simulink model "sim_battery_pack_simulink_18_11"  (R2021a)
settings: Solver=FixedStepAuto  StartTime=0.0  StopTime=3460.480  FixedStep=0.01  RelTol=1e-3
values from neighbouring files (symbols this model uses):
  Af = 1.4*1.6    (= 2.24)    [battery_pack_init_18_11.m]
  b = 0.002    [battery_pack_init_18_11.m]
  Batt_Eff = .98    (= 0.98)    [battery_pack_init_18_11.m]
  Batt_Ene_Cap = 7.37    [battery_pack_init_18_11.m]
  cd = 0.45    [battery_pack_init_18_11.m]
  dt = 0.01    [battery_pack_init_18_11.m]
  g = 9.81    [battery_pack_init_18_11.m]
  Gr = 5.75*.85    (= 4.8875)    [battery_pack_init_18_11.m]
  Grade = 7    [battery_pack_init_18_11.m]
  Ini_SOC = 100    [battery_pack_init_18_11.m]
  kappa = 0.1    [battery_pack_init_18_11.m]
  M = M_k+M_P    (= 445)    [battery_pack_init_18_11.m]
  M_Trq = T_m    [battery_pack_init_18_11.m]
  M_w = w_m    [battery_pack_init_18_11.m]
  Mot_Eff = .9    (= 0.9)    [battery_pack_init_18_11.m]
  mu = 0.016    [battery_pack_init_18_11.m]
  Np = 7    [battery_pack_init_18_11.m]
  Ns = 12    [battery_pack_init_18_11.m]
  Qgain = 1    [battery_pack_init_18_11.m]
  R0 = zeros(numpoles,1)    [battery_pack_init_18_11.m]
  R0Param = getParamESC('R0Param',T,cell_model)    [battery_pack_init_18_11.m]
  R_w = .3048/2    (= 0.1524)    [battery_pack_init_18_11.m]
  Re_spe_max = 50*5/18    (= 13.8888888889)    [battery_pack_init_18_11.m]
  Re_spe_min = 0*5/18    (= 0)    [battery_pack_init_18_11.m]
  rho = 1.225    [battery_pack_init_18_11.m]
  rt = .0008    (= 0.0008)    [battery_pack_init_18_11.m]
  T = 40    [battery_pack_init_18_11.m]
  T_MIDC = T_MIDC(1:72)    [battery_pack_init_18_11.m]
  Trans_Eff = .95    (= 0.95)    [battery_pack_init_18_11.m]
  V_MIDC = V_MIDC(1:72)    [battery_pack_init_18_11.m]
  Z0 = 0.75 + (1-0.75).*rand(1,Np)    [battery_pack_init_18_11.m]
undefined symbols (not defined in the file or in its folder): cell_model, FLbattery, gain, iload, sigbuilder_block, VMIDC
libraries: simulink x16, autolibshared x2, pid_lib x1, simulink_extras x1
(part 1 of 17)
settings Model: Creator=User  LastModifiedBy=User

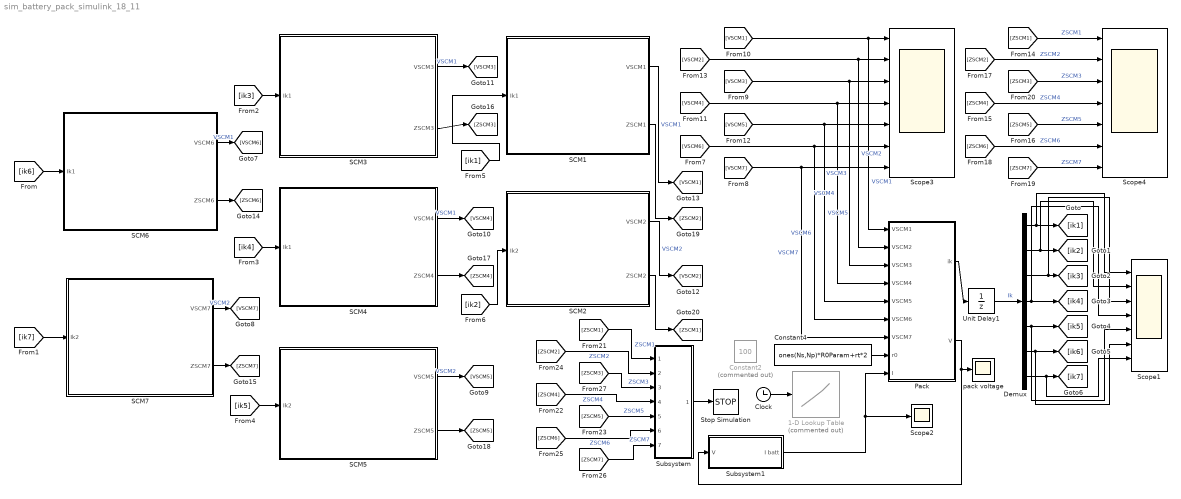
== system sim_battery_pack_simulink_18_11 ==
  1-D Lookup Table : Lookup_n-D  Commented=on  NumberOfTableDimensions=1  BreakpointsForDimension1=0:0.01:3460.480  Table=iload  InternalRulePriority=Speed  RndMeth=Simplest  InputSameDT=on
  Clock : Clock
  Constant2 : Constant  Commented=on  Value=100
  Constant4 : Constant  Value=ones(Ns,Np)*R0Param+rt*2
  Demux : Demux  Outputs=7
  Pack : MATLAB Function  TreatAsAtomicUnit=on
  SCM1 : Subsystem
  SCM2 : Subsystem
  SCM3 : Subsystem
  SCM4 : Subsystem
  SCM5 : Subsystem
  SCM6 : Subsystem
  SCM7 : Subsystem
  Scope1 : Scope  NumInputPorts=7
  Scope2 : Scope
  Scope3 : Scope  NumInputPorts=7
  Scope4 : Scope  NumInputPorts=7
  Stop Simulation : Stop
  Subsystem : Subsystem
  Subsystem1 : Subsystem
  Unit Delay1 : UnitDelay  SampleTime=-1  HasFrameUpgradeWarning=on
  pack voltage : Scope
  wires:
  Subsystem1/1(I batt) -> Pack/9(I), Scope2/1
  [VSCM1] -> Pack/1(VSCM1), Scope3/1  "VSCM1"
  [VSCM2] -> Scope3/2, Pack/2(VSCM2)  "VSCM2"
  Pack/1(ik) -> Unit Delay1/1
  Unit Delay1/1 -> Demux/1  "Ik"
  Constant4/1 -> Pack/8(r0)
  Clock/1 -> 1-D Lookup Table/1
  [VSCM3] -> Scope3/3, Pack/3(VSCM3)  "VSCM3"
  [VSCM4] -> Pack/4(VSCM4), Scope3/4  "VSCM4"
  [VSCM5] -> Pack/5(VSCM5), Scope3/5  "VSCM5"
  [VSCM6] -> Pack/6(VSCM6), Scope3/6  "VSCM6"
  [VSCM7] -> Scope3/7, Pack/7(VSCM7)  "VSCM7"
  [ik7] -> SCM7/1(Ik2)
  [ik6] -> SCM6/1(Ik1)
  [ik3] -> SCM3/1(Ik1)
  [ik4] -> SCM4/1(Ik1)
  [ik5] -> SCM5/1(Ik2)
  [ik2] -> SCM2/1(Ik2)
  [ik1] -> SCM1/1(Ik1)
  Demux/1 -> Scope1/1, [ik1]
  Demux/2 -> [ik2], Scope1/2
  Demux/3 -> Scope1/3, [ik3]
  Demux/4 -> [ik4], Scope1/4
  Demux/5 -> [ik5], Scope1/5
  Demux/6 -> [ik6], Scope1/6
  Demux/7 -> Scope1/7, [ik7]
  SCM6/1(VSCM6) -> [VSCM6]  "VSCM1"
  SCM7/1(VSCM7) -> [VSCM7]  "VSCM2"
  SCM1/1(VSCM1) -> [VSCM1]  "VSCM1"
  SCM2/1(VSCM2) -> [VSCM2]  "VSCM2"
  SCM5/1(VSCM5) -> [VSCM5]  "VSCM2"
  SCM4/1(VSCM4) -> [VSCM4]  "VSCM1"
  SCM3/1(VSCM3) -> [VSCM3]  "VSCM1"
  Pack/2(V) -> Subsystem1/1(V), pack voltage/1
  SCM6/2(ZSCM6) -> [ZSCM6]
  SCM7/2(ZSCM7) -> [ZSCM7]
  SCM3/2(ZSCM3) -> [ZSCM3]
  SCM4/2(ZSCM4) -> [ZSCM4]
  SCM5/2(ZSCM5) -> [ZSCM5]
  SCM1/2(ZSCM1) -> [ZSCM2]
  SCM2/2(ZSCM2) -> [ZSCM1]
  [ZSCM7] -> Scope4/7  "ZSCM7"
  [ZSCM6] -> Scope4/6  "ZSCM6"
  [ZSCM5] -> Scope4/5  "ZSCM5"
  [ZSCM4] -> Scope4/4  "ZSCM4"
  [ZSCM3] -> Scope4/3  "ZSCM3"
  [ZSCM2] -> Scope4/2  "ZSCM2"
  [ZSCM1] -> Scope4/1  "ZSCM1"
  [ZSCM2] -> Subsystem/2(ZSCM2)  "ZSCM2"
  [ZSCM4] -> Subsystem/4(ZSCM4)  "ZSCM4"
  [ZSCM6] -> Subsystem/6(ZSCM6)  "ZSCM6"
  [ZSCM1] -> Subsystem/1(ZSCM1)  "ZSCM1"
  [ZSCM3] -> Subsystem/3(ZSCM3)  "ZSCM3"
  [ZSCM5] -> Subsystem/5(ZSCM5)  "ZSCM5"
  [ZSCM7] -> Subsystem/7(ZSCM7)  "ZSCM7"
  Subsystem/1(STOP) -> Stop Simulation/1

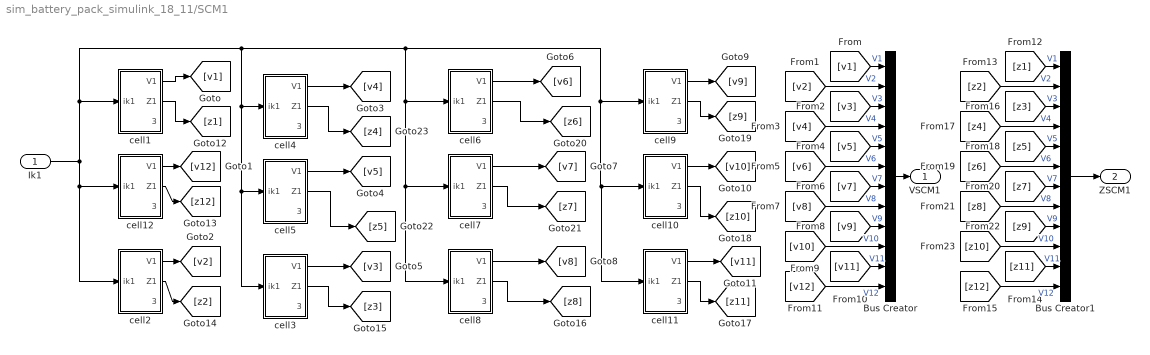
== system sim_battery_pack_simulink_18_11/SCM1 ==
  Ik1 : Inport
  Bus Creator : BusCreator  Inputs=12
  Bus Creator1 : BusCreator  Inputs=12
  cell1 : Subsystem
  cell10 : Subsystem
  cell11 : Subsystem
  cell12 : Subsystem
  cell2 : Subsystem
  cell3 : Subsystem
  cell4 : Subsystem
  cell5 : Subsystem
  cell6 : Subsystem
  cell7 : Subsystem
  cell8 : Subsystem
  cell9 : Subsystem
  VSCM1 : Outport
  ZSCM1 : Outport  Port=2
  wires:
  cell11/1(V1) -> [v11]
  cell8/1(V1) -> [v8]
  cell2/1(V1) -> [v2]
  cell1/1(V1) -> [v1]
  cell12/1(V1) -> [v12]
  cell7/1(V1) -> [v7]
  cell10/1(V1) -> [v10]
  Ik1/1 -> cell2/1(ik1), cell12/1(ik1), cell1/1(ik1), cell9/1(ik1), cell11/1(ik1), cell10/1(ik1), cell6/1(ik1), cell8/1(ik1), cell7/1(ik1), cell4/1(ik1), cell5/1(ik1), cell3/1(ik1)
  [v1] -> Bus Creator/1  "V1"
  [v2] -> Bus Creator/2  "V2"
  cell4/1(V1) -> [v4]
  cell5/1(V1) -> [v5]
  cell3/1(V1) -> [v3]
  cell6/1(V1) -> [v6]
  cell9/1(V1) -> [v9]
  [v3] -> Bus Creator/3  "V3"
  [v4] -> Bus Creator/4  "V4"
  [v5] -> Bus Creator/5  "V5"
  [v6] -> Bus Creator/6  "V6"
  [v7] -> Bus Creator/7  "V7"
  [v8] -> Bus Creator/8  "V8"
  [v9] -> Bus Creator/9  "V9"
  [v10] -> Bus Creator/10  "V10"
  [v11] -> Bus Creator/11  "V11"
  [v12] -> Bus Creator/12  "V12"
  Bus Creator/1 -> VSCM1/1
  cell1/2(Z1) -> [z1]
  cell12/2(Z1) -> [z12]
  cell2/2(Z1) -> [z2]
  cell8/2(Z1) -> [z8]
  cell11/2(Z1) -> [z11]
  cell10/2(Z1) -> [z10]
  cell9/2(Z1) -> [z9]
  cell6/2(Z1) -> [z6]
  cell7/2(Z1) -> [z7]
  cell3/2(Z1) -> [z3]
  cell5/2(Z1) -> [z5]
  cell4/2(Z1) -> [z4]
  Bus Creator1/1 -> ZSCM1/1
  [z12] -> Bus Creator1/12  "V12"
  [z11] -> Bus Creator1/11  "V11"
  [z10] -> Bus Creator1/10  "V10"
  [z9] -> Bus Creator1/9  "V9"
  [z8] -> Bus Creator1/8  "V8"
  [z7] -> Bus Creator1/7  "V7"
  [z6] -> Bus Creator1/6  "V6"
  [z5] -> Bus Creator1/5  "V5"
  [z4] -> Bus Creator1/4  "V4"
  [z3] -> Bus Creator1/3  "V3"
  [z2] -> Bus Creator1/2  "V2"
  [z1] -> Bus Creator1/1  "V1"

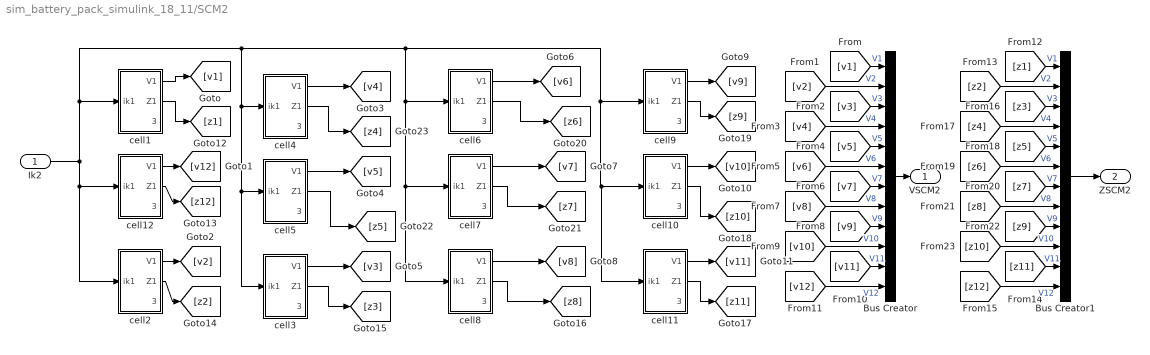
== system sim_battery_pack_simulink_18_11/SCM2 ==
  Ik2 : Inport
  Bus Creator : BusCreator  Inputs=12
  Bus Creator1 : BusCreator  Inputs=12
  cell1 : Subsystem
  cell10 : Subsystem
  cell11 : Subsystem
  cell12 : Subsystem
  cell2 : Subsystem
  cell3 : Subsystem
  cell4 : Subsystem
  cell5 : Subsystem
  cell6 : Subsystem
  cell7 : Subsystem
  cell8 : Subsystem
  cell9 : Subsystem
  VSCM2 : Outport
  ZSCM2 : Outport  Port=2
  wires:
  [z1] -> Bus Creator1/1  "V1"
  [z2] -> Bus Creator1/2  "V2"
  [z3] -> Bus Creator1/3  "V3"
  [z4] -> Bus Creator1/4  "V4"
  [z5] -> Bus Creator1/5  "V5"
  [z6] -> Bus Creator1/6  "V6"
  [z7] -> Bus Creator1/7  "V7"
  [z8] -> Bus Creator1/8  "V8"
  [z9] -> Bus Creator1/9  "V9"
  [z10] -> Bus Creator1/10  "V10"
  [z11] -> Bus Creator1/11  "V11"
  [z12] -> Bus Creator1/12  "V12"
  Bus Creator1/1 -> ZSCM2/1
  cell4/2(Z1) -> [z4]
  cell5/2(Z1) -> [z5]
  cell3/2(Z1) -> [z3]
  cell7/2(Z1) -> [z7]
  cell6/2(Z1) -> [z6]
  cell9/2(Z1) -> [z9]
  cell10/2(Z1) -> [z10]
  cell11/2(Z1) -> [z11]
  cell8/2(Z1) -> [z8]
  cell2/2(Z1) -> [z2]
  cell12/2(Z1) -> [z12]
  cell1/2(Z1) -> [z1]
  Bus Creator/1 -> VSCM2/1
  [v12] -> Bus Creator/12  "V12"
  [v11] -> Bus Creator/11  "V11"
  [v10] -> Bus Creator/10  "V10"
  [v9] -> Bus Creator/9  "V9"
  [v8] -> Bus Creator/8  "V8"
  [v7] -> Bus Creator/7  "V7"
  [v6] -> Bus Creator/6  "V6"
  [v5] -> Bus Creator/5  "V5"
  [v4] -> Bus Creator/4  "V4"
  [v3] -> Bus Creator/3  "V3"
  cell9/1(V1) -> [v9]
  cell6/1(V1) -> [v6]
  cell3/1(V1) -> [v3]
  cell5/1(V1) -> [v5]
  cell4/1(V1) -> [v4]
  [v2] -> Bus Creator/2  "V2"
  [v1] -> Bus Creator/1  "V1"
  Ik2/1 -> cell3/1(ik1), cell5/1(ik1), cell4/1(ik1), cell7/1(ik1), cell8/1(ik1), cell6/1(ik1), cell10/1(ik1), cell11/1(ik1), cell9/1(ik1), cell1/1(ik1), cell12/1(ik1), cell2/1(ik1)
  cell10/1(V1) -> [v10]
  cell7/1(V1) -> [v7]
  cell12/1(V1) -> [v12]
  cell1/1(V1) -> [v1]
  cell2/1(V1) -> [v2]
  cell8/1(V1) -> [v8]
  cell11/1(V1) -> [v11]

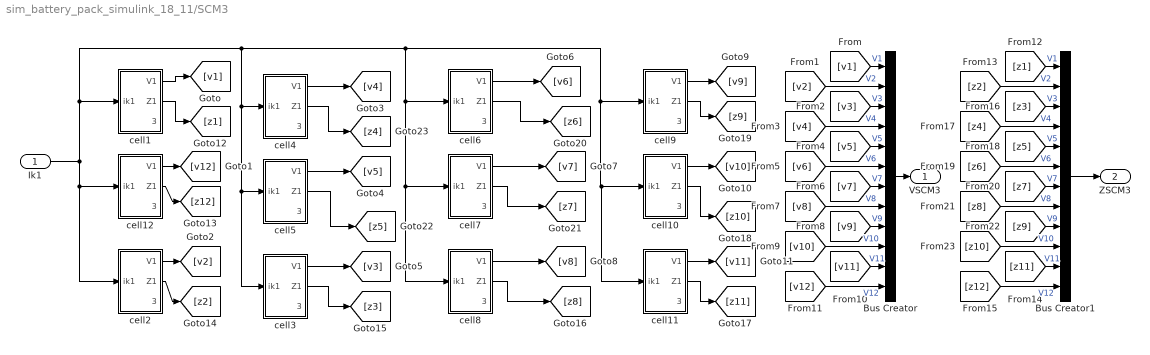
== system sim_battery_pack_simulink_18_11/SCM3 ==
  Ik1 : Inport
  Bus Creator : BusCreator  Inputs=12
  Bus Creator1 : BusCreator  Inputs=12
  cell1 : Subsystem
  cell10 : Subsystem
  cell11 : Subsystem
  cell12 : Subsystem
  cell2 : Subsystem
  cell3 : Subsystem
  cell4 : Subsystem
  cell5 : Subsystem
  cell6 : Subsystem
  cell7 : Subsystem
  cell8 : Subsystem
  cell9 : Subsystem
  VSCM3 : Outport
  ZSCM3 : Outport  Port=2
  wires:
  cell11/1(V1) -> [v11]
  cell8/1(V1) -> [v8]
  cell2/1(V1) -> [v2]
  cell1/1(V1) -> [v1]
  cell12/1(V1) -> [v12]
  cell7/1(V1) -> [v7]
  cell10/1(V1) -> [v10]
  Ik1/1 -> cell2/1(ik1), cell12/1(ik1), cell1/1(ik1), cell9/1(ik1), cell11/1(ik1), cell10/1(ik1), cell6/1(ik1), cell8/1(ik1), cell7/1(ik1), cell4/1(ik1), cell5/1(ik1), cell3/1(ik1)
  [v1] -> Bus Creator/1  "V1"
  [v2] -> Bus Creator/2  "V2"
  cell4/1(V1) -> [v4]
  cell5/1(V1) -> [v5]
  cell3/1(V1) -> [v3]
  cell6/1(V1) -> [v6]
  cell9/1(V1) -> [v9]
  [v3] -> Bus Creator/3  "V3"
  [v4] -> Bus Creator/4  "V4"
  [v5] -> Bus Creator/5  "V5"
  [v6] -> Bus Creator/6  "V6"
  [v7] -> Bus Creator/7  "V7"
  [v8] -> Bus Creator/8  "V8"
  [v9] -> Bus Creator/9  "V9"
  [v10] -> Bus Creator/10  "V10"
  [v11] -> Bus Creator/11  "V11"
  [v12] -> Bus Creator/12  "V12"
  Bus Creator/1 -> VSCM3/1
  cell1/2(Z1) -> [z1]
  cell12/2(Z1) -> [z12]
  cell2/2(Z1) -> [z2]
  cell8/2(Z1) -> [z8]
  cell11/2(Z1) -> [z11]
  cell10/2(Z1) -> [z10]
  cell9/2(Z1) -> [z9]
  cell6/2(Z1) -> [z6]
  cell7/2(Z1) -> [z7]
  cell3/2(Z1) -> [z3]
  cell5/2(Z1) -> [z5]
  cell4/2(Z1) -> [z4]
  Bus Creator1/1 -> ZSCM3/1
  [z12] -> Bus Creator1/12  "V12"
  [z11] -> Bus Creator1/11  "V11"
  [z10] -> Bus Creator1/10  "V10"
  [z9] -> Bus Creator1/9  "V9"
  [z8] -> Bus Creator1/8  "V8"
  [z7] -> Bus Creator1/7  "V7"
  [z6] -> Bus Creator1/6  "V6"
  [z5] -> Bus Creator1/5  "V5"
  [z4] -> Bus Creator1/4  "V4"
  [z3] -> Bus Creator1/3  "V3"
  [z2] -> Bus Creator1/2  "V2"
  [z1] -> Bus Creator1/1  "V1"

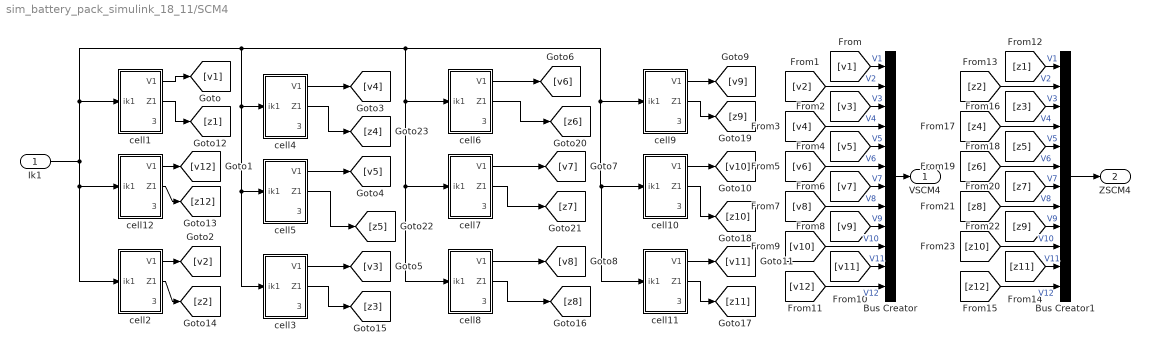
== system sim_battery_pack_simulink_18_11/SCM4 ==
  Ik1 : Inport
  Bus Creator : BusCreator  Inputs=12
  Bus Creator1 : BusCreator  Inputs=12
  cell1 : Subsystem
  cell10 : Subsystem
  cell11 : Subsystem
  cell12 : Subsystem
  cell2 : Subsystem
  cell3 : Subsystem
  cell4 : Subsystem
  cell5 : Subsystem
  cell6 : Subsystem
  cell7 : Subsystem
  cell8 : Subsystem
  cell9 : Subsystem
  VSCM4 : Outport
  ZSCM4 : Outport  Port=2
  wires:
  [z1] -> Bus Creator1/1  "V1"
  [z2] -> Bus Creator1/2  "V2"
  [z3] -> Bus Creator1/3  "V3"
  [z4] -> Bus Creator1/4  "V4"
  [z5] -> Bus Creator1/5  "V5"
  [z6] -> Bus Creator1/6  "V6"
  [z7] -> Bus Creator1/7  "V7"
  [z8] -> Bus Creator1/8  "V8"
  [z9] -> Bus Creator1/9  "V9"
  [z10] -> Bus Creator1/10  "V10"
  [z11] -> Bus Creator1/11  "V11"
  [z12] -> Bus Creator1/12  "V12"
  Bus Creator1/1 -> ZSCM4/1
  cell4/2(Z1) -> [z4]
  cell5/2(Z1) -> [z5]
  cell3/2(Z1) -> [z3]
  cell7/2(Z1) -> [z7]
  cell6/2(Z1) -> [z6]
  cell9/2(Z1) -> [z9]
  cell10/2(Z1) -> [z10]
  cell11/2(Z1) -> [z11]
  cell8/2(Z1) -> [z8]
  cell2/2(Z1) -> [z2]
  cell12/2(Z1) -> [z12]
  cell1/2(Z1) -> [z1]
  Bus Creator/1 -> VSCM4/1
  [v12] -> Bus Creator/12  "V12"
  [v11] -> Bus Creator/11  "V11"
  [v10] -> Bus Creator/10  "V10"
  [v9] -> Bus Creator/9  "V9"
  [v8] -> Bus Creator/8  "V8"
  [v7] -> Bus Creator/7  "V7"
  [v6] -> Bus Creator/6  "V6"
  [v5] -> Bus Creator/5  "V5"
  [v4] -> Bus Creator/4  "V4"
  [v3] -> Bus Creator/3  "V3"
  cell9/1(V1) -> [v9]
  cell6/1(V1) -> [v6]
  cell3/1(V1) -> [v3]
  cell5/1(V1) -> [v5]
  cell4/1(V1) -> [v4]
  [v2] -> Bus Creator/2  "V2"
  [v1] -> Bus Creator/1  "V1"
  Ik1/1 -> cell3/1(ik1), cell5/1(ik1), cell4/1(ik1), cell7/1(ik1), cell8/1(ik1), cell6/1(ik1), cell10/1(ik1), cell11/1(ik1), cell9/1(ik1), cell1/1(ik1), cell12/1(ik1), cell2/1(ik1)
  cell10/1(V1) -> [v10]
  cell7/1(V1) -> [v7]
  cell12/1(V1) -> [v12]
  cell1/1(V1) -> [v1]
  cell2/1(V1) -> [v2]
  cell8/1(V1) -> [v8]
  cell11/1(V1) -> [v11]

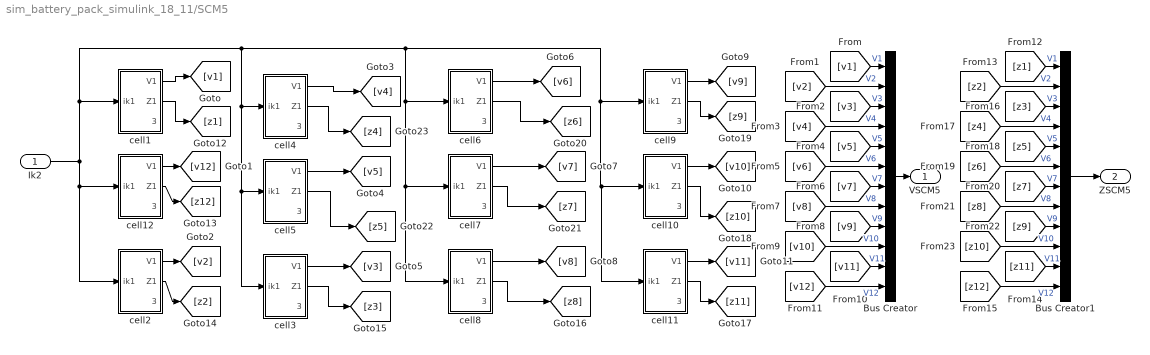
== system sim_battery_pack_simulink_18_11/SCM5 ==
  Ik2 : Inport
  Bus Creator : BusCreator  Inputs=12
  Bus Creator1 : BusCreator  Inputs=12
  cell1 : Subsystem
  cell10 : Subsystem
  cell11 : Subsystem
  cell12 : Subsystem
  cell2 : Subsystem
  cell3 : Subsystem
  cell4 : Subsystem
  cell5 : Subsystem
  cell6 : Subsystem
  cell7 : Subsystem
  cell8 : Subsystem
  cell9 : Subsystem
  VSCM5 : Outport
  ZSCM5 : Outport  Port=2
  wires:
  [z1] -> Bus Creator1/1  "V1"
  [z2] -> Bus Creator1/2  "V2"
  [z3] -> Bus Creator1/3  "V3"
  [z4] -> Bus Creator1/4  "V4"
  [z5] -> Bus Creator1/5  "V5"
  [z6] -> Bus Creator1/6  "V6"
  [z7] -> Bus Creator1/7  "V7"
  [z8] -> Bus Creator1/8  "V8"
  [z9] -> Bus Creator1/9  "V9"
  [z10] -> Bus Creator1/10  "V10"
  [z11] -> Bus Creator1/11  "V11"
  [z12] -> Bus Creator1/12  "V12"
  Bus Creator1/1 -> ZSCM5/1
  cell4/2(Z1) -> [z4]
  cell5/2(Z1) -> [z5]
  cell3/2(Z1) -> [z3]
  cell7/2(Z1) -> [z7]
  cell6/2(Z1) -> [z6]
  cell9/2(Z1) -> [z9]
  cell10/2(Z1) -> [z10]
  cell11/2(Z1) -> [z11]
  cell8/2(Z1) -> [z8]
  cell2/2(Z1) -> [z2]
  cell12/2(Z1) -> [z12]
  cell1/2(Z1) -> [z1]
  Bus Creator/1 -> VSCM5/1
  [v12] -> Bus Creator/12  "V12"
  [v11] -> Bus Creator/11  "V11"
  [v10] -> Bus Creator/10  "V10"
  [v9] -> Bus Creator/9  "V9"
  [v8] -> Bus Creator/8  "V8"
  [v7] -> Bus Creator/7  "V7"
  [v6] -> Bus Creator/6  "V6"
  [v5] -> Bus Creator/5  "V5"
  [v4] -> Bus Creator/4  "V4"
  [v3] -> Bus Creator/3  "V3"
  cell9/1(V1) -> [v9]
  cell6/1(V1) -> [v6]
  cell3/1(V1) -> [v3]
  cell5/1(V1) -> [v5]
  cell4/1(V1) -> [v4]
  [v2] -> Bus Creator/2  "V2"
  [v1] -> Bus Creator/1  "V1"
  Ik2/1 -> cell3/1(ik1), cell5/1(ik1), cell4/1(ik1), cell7/1(ik1), cell8/1(ik1), cell6/1(ik1), cell10/1(ik1), cell11/1(ik1), cell9/1(ik1), cell1/1(ik1), cell12/1(ik1), cell2/1(ik1)
  cell10/1(V1) -> [v10]
  cell7/1(V1) -> [v7]
  cell12/1(V1) -> [v12]
  cell1/1(V1) -> [v1]
  cell2/1(V1) -> [v2]
  cell8/1(V1) -> [v8]
  cell11/1(V1) -> [v11]

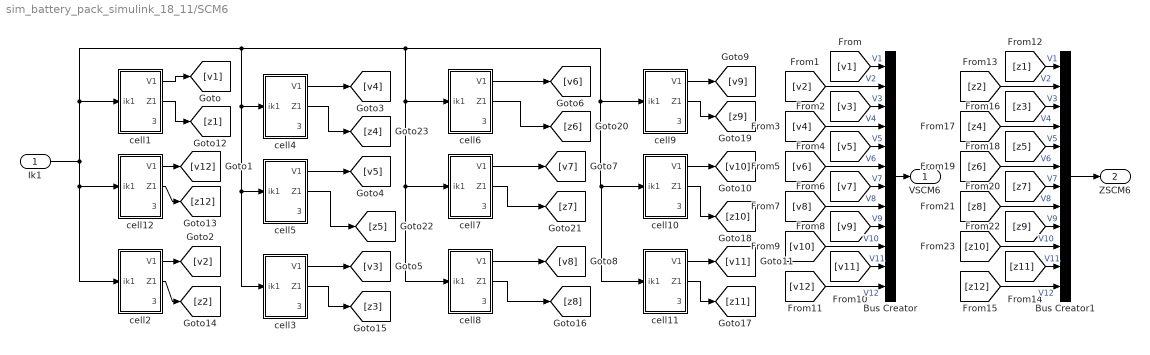
== system sim_battery_pack_simulink_18_11/SCM6 ==
  Ik1 : Inport
  Bus Creator : BusCreator  Inputs=12
  Bus Creator1 : BusCreator  Inputs=12
  cell1 : Subsystem
  cell10 : Subsystem
  cell11 : Subsystem
  cell12 : Subsystem
  cell2 : Subsystem
  cell3 : Subsystem
  cell4 : Subsystem
  cell5 : Subsystem
  cell6 : Subsystem
  cell7 : Subsystem
  cell8 : Subsystem
  cell9 : Subsystem
  VSCM6 : Outport
  ZSCM6 : Outport  Port=2
  wires:
  [z1] -> Bus Creator1/1  "V1"
  [z2] -> Bus Creator1/2  "V2"
  [z3] -> Bus Creator1/3  "V3"
  [z4] -> Bus Creator1/4  "V4"
  [z5] -> Bus Creator1/5  "V5"
  [z6] -> Bus Creator1/6  "V6"
  [z7] -> Bus Creator1/7  "V7"
  [z8] -> Bus Creator1/8  "V8"
  [z9] -> Bus Creator1/9  "V9"
  [z10] -> Bus Creator1/10  "V10"
  [z11] -> Bus Creator1/11  "V11"
  [z12] -> Bus Creator1/12  "V12"
  Bus Creator1/1 -> ZSCM6/1
  cell4/2(Z1) -> [z4]
  cell5/2(Z1) -> [z5]
  cell3/2(Z1) -> [z3]
  cell7/2(Z1) -> [z7]
  cell6/2(Z1) -> [z6]
  cell9/2(Z1) -> [z9]
  cell10/2(Z1) -> [z10]
  cell11/2(Z1) -> [z11]
  cell8/2(Z1) -> [z8]
  cell2/2(Z1) -> [z2]
  cell12/2(Z1) -> [z12]
  cell1/2(Z1) -> [z1]
  Bus Creator/1 -> VSCM6/1
  [v12] -> Bus Creator/12  "V12"
  [v11] -> Bus Creator/11  "V11"
  [v10] -> Bus Creator/10  "V10"
  [v9] -> Bus Creator/9  "V9"
  [v8] -> Bus Creator/8  "V8"
  [v7] -> Bus Creator/7  "V7"
  [v6] -> Bus Creator/6  "V6"
  [v5] -> Bus Creator/5  "V5"
  [v4] -> Bus Creator/4  "V4"
  [v3] -> Bus Creator/3  "V3"
  cell9/1(V1) -> [v9]
  cell6/1(V1) -> [v6]
  cell3/1(V1) -> [v3]
  cell5/1(V1) -> [v5]
  cell4/1(V1) -> [v4]
  [v2] -> Bus Creator/2  "V2"
  [v1] -> Bus Creator/1  "V1"
  Ik1/1 -> cell3/1(ik1), cell5/1(ik1), cell4/1(ik1), cell7/1(ik1), cell8/1(ik1), cell6/1(ik1), cell10/1(ik1), cell11/1(ik1), cell9/1(ik1), cell1/1(ik1), cell12/1(ik1), cell2/1(ik1)
  cell10/1(V1) -> [v10]
  cell7/1(V1) -> [v7]
  cell12/1(V1) -> [v12]
  cell1/1(V1) -> [v1]
  cell2/1(V1) -> [v2]
  cell8/1(V1) -> [v8]
  cell11/1(V1) -> [v11]

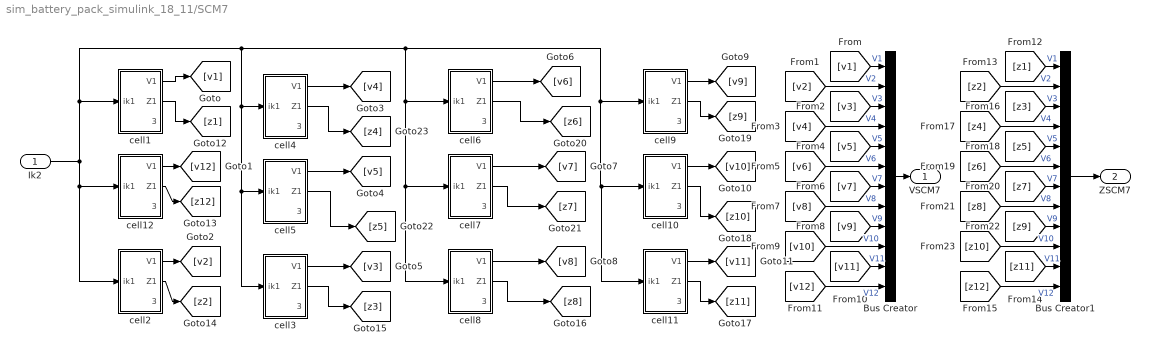
== system sim_battery_pack_simulink_18_11/SCM7 ==
  Ik2 : Inport
  Bus Creator : BusCreator  Inputs=12
  Bus Creator1 : BusCreator  Inputs=12
  cell1 : Subsystem
  cell10 : Subsystem
  cell11 : Subsystem
  cell12 : Subsystem
  cell2 : Subsystem
  cell3 : Subsystem
  cell4 : Subsystem
  cell5 : Subsystem
  cell6 : Subsystem
  cell7 : Subsystem
  cell8 : Subsystem
  cell9 : Subsystem
  VSCM7 : Outport
  ZSCM7 : Outport  Port=2
  wires:
  cell11/1(V1) -> [v11]
  cell8/1(V1) -> [v8]
  cell2/1(V1) -> [v2]
  cell1/1(V1) -> [v1]
  cell12/1(V1) -> [v12]
  cell7/1(V1) -> [v7]
  cell10/1(V1) -> [v10]
  Ik2/1 -> cell2/1(ik1), cell12/1(ik1), cell1/1(ik1), cell9/1(ik1), cell11/1(ik1), cell10/1(ik1), cell6/1(ik1), cell8/1(ik1), cell7/1(ik1), cell4/1(ik1), cell5/1(ik1), cell3/1(ik1)
  [v1] -> Bus Creator/1  "V1"
  [v2] -> Bus Creator/2  "V2"
  cell4/1(V1) -> [v4]
  cell5/1(V1) -> [v5]
  cell3/1(V1) -> [v3]
  cell6/1(V1) -> [v6]
  cell9/1(V1) -> [v9]
  [v3] -> Bus Creator/3  "V3"
  [v4] -> Bus Creator/4  "V4"
  [v5] -> Bus Creator/5  "V5"
  [v6] -> Bus Creator/6  "V6"
  [v7] -> Bus Creator/7  "V7"
  [v8] -> Bus Creator/8  "V8"
  [v9] -> Bus Creator/9  "V9"
  [v10] -> Bus Creator/10  "V10"
  [v11] -> Bus Creator/11  "V11"
  [v12] -> Bus Creator/12  "V12"
  Bus Creator/1 -> VSCM7/1
  cell1/2(Z1) -> [z1]
  cell12/2(Z1) -> [z12]
  cell2/2(Z1) -> [z2]
  cell8/2(Z1) -> [z8]
  cell11/2(Z1) -> [z11]
  cell10/2(Z1) -> [z10]
  cell9/2(Z1) -> [z9]
  cell6/2(Z1) -> [z6]
  cell7/2(Z1) -> [z7]
  cell3/2(Z1) -> [z3]
  cell5/2(Z1) -> [z5]
  cell4/2(Z1) -> [z4]
  Bus Creator1/1 -> ZSCM7/1
  [z12] -> Bus Creator1/12  "V12"
  [z11] -> Bus Creator1/11  "V11"
  [z10] -> Bus Creator1/10  "V10"
  [z9] -> Bus Creator1/9  "V9"
  [z8] -> Bus Creator1/8  "V8"
  [z7] -> Bus Creator1/7  "V7"
  [z6] -> Bus Creator1/6  "V6"
  [z5] -> Bus Creator1/5  "V5"
  [z4] -> Bus Creator1/4  "V4"
  [z3] -> Bus Creator1/3  "V3"
  [z2] -> Bus Creator1/2  "V2"
  [z1] -> Bus Creator1/1  "V1"

== system sim_battery_pack_simulink_18_11/Subsystem ==
  ZSCM1 : Inport
  ZSCM2 : Inport  Port=2
  ZSCM3 : Inport  Port=3
  ZSCM4 : Inport  Port=4
  ZSCM5 : Inport  Port=5
  ZSCM6 : Inport  Port=6
  ZSCM7 : Inport  Port=7
  Bus Creator : BusCreator  Inputs=7
  Compare To Constant : simulink/Logic and Bit Operations/Compare To Constant  relop=<=  const=0.05  OutDataTypeStr=boolean
  Display : Display
  Min of Elements : MinMax
  STOP : Outport
  wires:
  ZSCM1/1 -> Bus Creator/1
  ZSCM2/1 -> Bus Creator/2
  ZSCM3/1 -> Bus Creator/3
  ZSCM4/1 -> Bus Creator/4
  ZSCM5/1 -> Bus Creator/5
  ZSCM6/1 -> Bus Creator/6
  ZSCM7/1 -> Bus Creator/7
  Bus Creator/1 -> Display/1, Min of Elements/1
  Min of Elements/1 -> Compare To Constant/1
  Compare To Constant/1 -> STOP/1

== system sim_battery_pack_simulink_18_11/Subsystem1 ==
  V : Inport
  Battery1 : Subsystem
      settings: PortSchema="{\"entries\":[{\"content\":{\"sides\":[{\"content\":{\"connectorIds\":[\"Out4\",\"In1\"]},\"type\":\"ConnectorPlacement.EquallySpacedRectSide\",\"uuid\":\"95f9873b-fe01-4ff7-a5ab-aada3bc95a03\"},{\"content\":{\"connectorIds\":[\"Out1\",\"In2\",\"Out2\",\"Out3\"],\"side\":\"RIGHT\"},\"type\":\"ConnectorPlacement.EquallySpacedRectSide\",\"uuid\":\"b4897c1e-778c-4bc7-a7f1-163b7f4cdad4\"},{\"content\":{\"connectorIds\":[],\"side\":\"TOP\"},\"type\":\"ConnectorPlacement.EquallySpacedRectSide\",\"uuid\":\"a4f74249-cbee-46b9-95a1-ffe2d651d1aa\"}]},\"type\":\"ConnectorPlacement.EquallySpacedConnector\",\"uuid\":\"65519a53-4300-47bd-84a6-9cdab8c1658d\"}],\"packageUris\":[\"http://schema.mathworks.com/mf0/Connector/R2020b\"],\"version\":\"1.0\"}"
  Constant3 : Constant  Value=7.37
  Constant4 : Constant
  Controller : Subsystem
      settings: PortSchema="{\"entries\":[{\"content\":{\"sides\":[{\"content\":{\"connectorIds\":[\"In1\",\"In2\",\"In3\"]},\"type\":\"ConnectorPlacement.EquallySpacedRectSide\",\"uuid\":\"7181f2fb-814d-454b-bbdd-5a6429464cde\"},{\"content\":{\"connectorIds\":[\"Out1\",\"In6\",\"Out2\"],\"side\":\"RIGHT\"},\"type\":\"ConnectorPlacement.EquallySpacedRectSide\",\"uuid\":\"9f09df5c-a21b-4dbe-b9f4-fd639a3fc7b6\"},{\"content\":{\"connectorIds\":[\"In4\",\"In5\"],\"side\":\"TOP\"},\"type\":\"ConnectorPlacement.EquallySpacedRectSide\",\"uuid\":\"cea066f6-5d29-4bfe-a52b-88d077042081\"}]},\"type\":\"ConnectorPlacement.EquallySpacedConnector\",\"uuid\":\"89d9cb73-964c-472c-86a0-f36e993decee\"}],\"packageUris\":[\"http://schema.mathworks.com/mf0/Connector/R2020b\"],\"version\":\"1.0\"}"
  Display2 : Display
  Divide : Product  Inputs=*/
  Driver : Subsystem
  Motor : Subsystem
  Product1 : Product
  Scope : Scope
  Scope1 : Scope  NumInputPorts=2
  Subtract : Sum  Inputs=+-
  Transmission : Subsystem
      settings: PortSchema="{\"entries\":[{\"content\":{\"sides\":[{\"content\":{\"connectorIds\":[\"In1\",\"Out2\"]},\"type\":\"ConnectorPlacement.EquallySpacedRectSide\",\"uuid\":\"6a60ea79-1d6a-43be-8c6e-faa96b9426ae\"},{\"content\":{\"connectorIds\":[\"Out1\",\"In2\"],\"side\":\"RIGHT\"},\"type\":\"ConnectorPlacement.EquallySpacedRectSide\",\"uuid\":\"ce7e119a-d2f4-42be-b472-f935cef86375\"},{\"content\":{\"connectorIds\":[],\"side\":\"TOP\"},\"type\":\"ConnectorPlacement.EquallySpacedRectSide\",\"uuid\":\"7967fcd3-5be4-4a26-8ccb-3cce446b495a\"}]},\"type\":\"ConnectorPlacement.EquallySpacedConnector\",\"uuid\":\"10659099-893a-4c78-98f4-a4e8ec8b982a\"}],\"packageUris\":[\"http://schema.mathworks.com/mf0/Connector/R2020b\"],\"version\":\"1.0\"}"
  Vehicle Dynamics : Subsystem
      settings: PortSchema="{\"entries\":[{\"content\":{\"sides\":[{\"content\":{\"connectorIds\":[\"In1\",\"Out3\",\"Out4\",\"In2\"]},\"type\":\"ConnectorPlacement.EquallySpacedRectSide\",\"uuid\":\"6a60ea79-1d6a-43be-8c6e-faa96b9426ae\"},{\"content\":{\"connectorIds\":[\"Out1\"],\"side\":\"RIGHT\"},\"type\":\"ConnectorPlacement.EquallySpacedRectSide\",\"uuid\":\"ce7e119a-d2f4-42be-b472-f935cef86375\"},{\"content\":{\"connectorIds\":[\"Out2\"],\"side\":\"TOP\"},\"type\":\"ConnectorPlacement.EquallySpacedRectSide\",\"uuid\":\"7967fcd3-5be4-4a26-8ccb-3cce446b495a\"}]},\"type\":\"ConnectorPlacement.EquallySpacedConnector\",\"uuid\":\"10659099-893a-4c78-98f4-a4e8ec8b982a\"}],\"packageUris\":[\"http://schema.mathworks.com/mf0/Connector/R2020b\"],\"version\":\"1.0\"}"
  Vehicle Monitoring : Subsystem  Commented=on
  km : Display
  kwhr/km : Display
  I batt : Outport
  tag scope: Soc=global
  wires:
  Product1/1 -> Divide/1
  Battery1/1(SOC) -> [Soc], Scope/1, Display2/1, Subtract/2
  Controller/1(TrqCmd) -> Motor/1(TrqCmd)
  Subtract/1 -> Product1/2
  Constant4/1 -> Subtract/1
  Motor/2(Mtr_trq) -> Transmission/1(MtrTrq)
  Vehicle Dynamics/4(VKm/h) -> Scope1/2
  Battery1/3(Regen_Pow_Lim) -> Controller/5(Regen_Lim)
  Divide/1 -> kwhr/km/1
  Driver/3(Vref) -> Scope1/1
  Driver/2(DecelCmd) -> Controller/2(Brake)
  Motor/1(Batt_Pow_Cons) -> Battery1/1(Battery power)
  Vehicle Dynamics/2(Dis) -> Divide/2, km/1
  Vehicle Dynamics/1(VehSpd) -> Controller/3(VehSpd), Driver/1(VelFdbk)
  Battery1/2(Draw_Pow_Lim) -> Controller/4(Draw_Lim)
  Transmission/1(AxleTrq) -> Vehicle Dynamics/1(AxleTrq)
  Controller/2(BrkForce) -> Vehicle Dynamics/2(BrakeForce)
  Driver/1(AccelCmd) -> Controller/1(AccelCmd)
  Transmission/2(MtrSpd) -> Controller/6(MtrSpd), Motor/2(MtrSpd)
  Vehicle Dynamics/3(AxleSpd) -> Transmission/2(AxleSpd)
  Constant3/1 -> Product1/1
  Battery1/4(I batt) -> I batt/1
  V/1 -> Battery1/2(V)

== system sim_battery_pack_simulink_18_11/SCM1/cell1 ==
  ik1 : Inport
  Constant : Constant  Value=R0
  Constant1 : Constant  Value=dt
  Constant2 : Constant  Value=T
  States : Scope  NumInputPorts=2
  Unit Delay : UnitDelay  InitialCondition=Z0(1,1)  SampleTime=-1  HasFrameUpgradeWarning=on
  Unit Delay1 : UnitDelay  SampleTime=-1  HasFrameUpgradeWarning=on
  Voltage : Scope  NumInputPorts=2
  cell_model : MATLAB Function  TreatAsAtomicUnit=on
  V1 : Outport
  Z1 : Outport  Port=2
  irc1 : Outport  Port=3
  wires:
  cell_model/4(OCV) -> Voltage/2
  ik1/1 -> cell_model/6(ik)
  cell_model/3(zkc) -> Z1/1, Unit Delay/1, States/1
  cell_model/1(vk) -> V1/1, Voltage/1
  Constant1/1 -> cell_model/2(deltaT)
  Constant2/1 -> cell_model/1(T)
  Unit Delay/1 -> cell_model/4(zkp)
  cell_model/2(irkc) -> irc1/1, Unit Delay1/1, States/2
  Unit Delay1/1 -> cell_model/5(irkp)
  Constant/1 -> cell_model/3(iR0)

== system sim_battery_pack_simulink_18_11/SCM1/cell10 ==
  ik1 : Inport
  Constant : Constant  Value=R0
  Constant1 : Constant  Value=dt
  Constant2 : Constant  Value=T
  States : Scope  NumInputPorts=2
  Unit Delay : UnitDelay  InitialCondition=Z0(10,1)  SampleTime=-1  HasFrameUpgradeWarning=on
  Unit Delay1 : UnitDelay  SampleTime=-1  HasFrameUpgradeWarning=on
  Voltage : Scope  NumInputPorts=2
  cell_model : MATLAB Function  TreatAsAtomicUnit=on
  V1 : Outport
  Z1 : Outport  Port=2
  irc1 : Outport  Port=3
  wires:
  cell_model/4(OCV) -> Voltage/2
  ik1/1 -> cell_model/6(ik)
  cell_model/3(zkc) -> Z1/1, Unit Delay/1, States/1
  cell_model/1(vk) -> V1/1, Voltage/1
  Constant1/1 -> cell_model/2(deltaT)
  Constant2/1 -> cell_model/1(T)
  Unit Delay/1 -> cell_model/4(zkp)
  cell_model/2(irkc) -> irc1/1, Unit Delay1/1, States/2
  Unit Delay1/1 -> cell_model/5(irkp)
  Constant/1 -> cell_model/3(iR0)

== system sim_battery_pack_simulink_18_11/SCM1/cell11 ==
  ik1 : Inport
  Constant : Constant  Value=R0
  Constant1 : Constant  Value=dt
  Constant2 : Constant  Value=T
  States : Scope  NumInputPorts=2
  Unit Delay : UnitDelay  InitialCondition=Z0(11,1)  SampleTime=-1  HasFrameUpgradeWarning=on
  Unit Delay1 : UnitDelay  SampleTime=-1  HasFrameUpgradeWarning=on
  Voltage : Scope  NumInputPorts=2
  cell_model : MATLAB Function  TreatAsAtomicUnit=on
  V1 : Outport
  Z1 : Outport  Port=2
  irc1 : Outport  Port=3
  wires:
  Constant/1 -> cell_model/3(iR0)
  Unit Delay1/1 -> cell_model/5(irkp)
  cell_model/2(irkc) -> States/2, Unit Delay1/1, irc1/1
  Unit Delay/1 -> cell_model/4(zkp)
  Constant2/1 -> cell_model/1(T)
  Constant1/1 -> cell_model/2(deltaT)
  cell_model/1(vk) -> Voltage/1, V1/1
  cell_model/3(zkc) -> States/1, Unit Delay/1, Z1/1
  ik1/1 -> cell_model/6(ik)
  cell_model/4(OCV) -> Voltage/2

== system sim_battery_pack_simulink_18_11/SCM1/cell12 ==
  ik1 : Inport
  Constant : Constant  Value=R0
  Constant1 : Constant  Value=dt
  Constant2 : Constant  Value=T
  States : Scope  NumInputPorts=2
  Unit Delay : UnitDelay  InitialCondition=Z0(12,1)  SampleTime=-1  HasFrameUpgradeWarning=on
  Unit Delay1 : UnitDelay  SampleTime=-1  HasFrameUpgradeWarning=on
  Voltage : Scope  NumInputPorts=2
  cell_model : MATLAB Function  TreatAsAtomicUnit=on
  V1 : Outport
  Z1 : Outport  Port=2
  irc1 : Outport  Port=3
  wires:
  Constant/1 -> cell_model/3(iR0)
  Unit Delay1/1 -> cell_model/5(irkp)
  cell_model/2(irkc) -> States/2, Unit Delay1/1, irc1/1
  Unit Delay/1 -> cell_model/4(zkp)
  Constant2/1 -> cell_model/1(T)
  Constant1/1 -> cell_model/2(deltaT)
  cell_model/1(vk) -> Voltage/1, V1/1
  cell_model/3(zkc) -> States/1, Unit Delay/1, Z1/1
  ik1/1 -> cell_model/6(ik)
  cell_model/4(OCV) -> Voltage/2

== system sim_battery_pack_simulink_18_11/SCM1/cell2 ==
  ik1 : Inport
  Constant : Constant  Value=R0
  Constant1 : Constant  Value=dt
  Constant2 : Constant  Value=T
  States : Scope  NumInputPorts=2
  Unit Delay : UnitDelay  InitialCondition=Z0(2,1)  SampleTime=-1  HasFrameUpgradeWarning=on
  Unit Delay1 : UnitDelay  SampleTime=-1  HasFrameUpgradeWarning=on
  Voltage : Scope  NumInputPorts=2
  cell_model : MATLAB Function  TreatAsAtomicUnit=on
  V1 : Outport
  Z1 : Outport  Port=2
  irc1 : Outport  Port=3
  wires:
  cell_model/4(OCV) -> Voltage/2
  ik1/1 -> cell_model/6(ik)
  cell_model/3(zkc) -> Z1/1, Unit Delay/1, States/1
  cell_model/1(vk) -> V1/1, Voltage/1
  Constant1/1 -> cell_model/2(deltaT)
  Constant2/1 -> cell_model/1(T)
  Unit Delay/1 -> cell_model/4(zkp)
  cell_model/2(irkc) -> irc1/1, Unit Delay1/1, States/2
  Unit Delay1/1 -> cell_model/5(irkp)
  Constant/1 -> cell_model/3(iR0)

== system sim_battery_pack_simulink_18_11/SCM1/cell3 ==
  ik1 : Inport
  Constant : Constant  Value=R0
  Constant1 : Constant  Value=dt
  Constant2 : Constant  Value=T
  States : Scope  NumInputPorts=2
  Unit Delay : UnitDelay  InitialCondition=Z0(3,1)  SampleTime=-1  HasFrameUpgradeWarning=on
  Unit Delay1 : UnitDelay  SampleTime=-1  HasFrameUpgradeWarning=on
  Voltage : Scope  NumInputPorts=2
  cell_model : MATLAB Function  TreatAsAtomicUnit=on
  V1 : Outport
  Z1 : Outport  Port=2
  irc1 : Outport  Port=3
  wires:
  Constant/1 -> cell_model/3(iR0)
  Unit Delay1/1 -> cell_model/5(irkp)
  cell_model/2(irkc) -> States/2, Unit Delay1/1, irc1/1
  Unit Delay/1 -> cell_model/4(zkp)
  Constant2/1 -> cell_model/1(T)
  Constant1/1 -> cell_model/2(deltaT)
  cell_model/1(vk) -> Voltage/1, V1/1
  cell_model/3(zkc) -> States/1, Unit Delay/1, Z1/1
  ik1/1 -> cell_model/6(ik)
  cell_model/4(OCV) -> Voltage/2

== system sim_battery_pack_simulink_18_11/SCM1/cell4 ==
  ik1 : Inport
  Constant : Constant  Value=R0
  Constant1 : Constant  Value=dt
  Constant2 : Constant  Value=T
  States : Scope  NumInputPorts=2
  Unit Delay : UnitDelay  InitialCondition=Z0(4,1)  SampleTime=-1  HasFrameUpgradeWarning=on
  Unit Delay1 : UnitDelay  SampleTime=-1  HasFrameUpgradeWarning=on
  Voltage : Scope  NumInputPorts=2
  cell_model : MATLAB Function  TreatAsAtomicUnit=on
  V1 : Outport
  Z1 : Outport  Port=2
  irc1 : Outport  Port=3
  wires:
  Constant/1 -> cell_model/3(iR0)
  Unit Delay1/1 -> cell_model/5(irkp)
  cell_model/2(irkc) -> States/2, Unit Delay1/1, irc1/1
  Unit Delay/1 -> cell_model/4(zkp)
  Constant2/1 -> cell_model/1(T)
  Constant1/1 -> cell_model/2(deltaT)
  cell_model/1(vk) -> Voltage/1, V1/1
  cell_model/3(zkc) -> States/1, Unit Delay/1, Z1/1
  ik1/1 -> cell_model/6(ik)
  cell_model/4(OCV) -> Voltage/2

== system sim_battery_pack_simulink_18_11/SCM1/cell5 ==
  ik1 : Inport
  Constant : Constant  Value=R0
  Constant1 : Constant  Value=dt
  Constant2 : Constant  Value=T
  States : Scope  NumInputPorts=2
  Unit Delay : UnitDelay  InitialCondition=Z0(5,1)  SampleTime=-1  HasFrameUpgradeWarning=on
  Unit Delay1 : UnitDelay  SampleTime=-1  HasFrameUpgradeWarning=on
  Voltage : Scope  NumInputPorts=2
  cell_model : MATLAB Function  TreatAsAtomicUnit=on
  V1 : Outport
  Z1 : Outport  Port=2
  irc1 : Outport  Port=3
  wires:
  cell_model/4(OCV) -> Voltage/2
  ik1/1 -> cell_model/6(ik)
  cell_model/3(zkc) -> Z1/1, Unit Delay/1, States/1
  cell_model/1(vk) -> V1/1, Voltage/1
  Constant1/1 -> cell_model/2(deltaT)
  Constant2/1 -> cell_model/1(T)
  Unit Delay/1 -> cell_model/4(zkp)
  cell_model/2(irkc) -> irc1/1, Unit Delay1/1, States/2
  Unit Delay1/1 -> cell_model/5(irkp)
  Constant/1 -> cell_model/3(iR0)

== system sim_battery_pack_simulink_18_11/SCM1/cell6 ==
  ik1 : Inport
  Constant : Constant  Value=R0
  Constant1 : Constant  Value=dt
  Constant2 : Constant  Value=T
  States : Scope  NumInputPorts=2
  Unit Delay : UnitDelay  InitialCondition=Z0(6,1)  SampleTime=-1  HasFrameUpgradeWarning=on
  Unit Delay1 : UnitDelay  SampleTime=-1  HasFrameUpgradeWarning=on
  Voltage : Scope  NumInputPorts=2
  cell_model : MATLAB Function  TreatAsAtomicUnit=on
  V1 : Outport
  Z1 : Outport  Port=2
  irc1 : Outport  Port=3
  wires:
  cell_model/4(OCV) -> Voltage/2
  ik1/1 -> cell_model/6(ik)
  cell_model/3(zkc) -> Z1/1, Unit Delay/1, States/1
  cell_model/1(vk) -> V1/1, Voltage/1
  Constant1/1 -> cell_model/2(deltaT)
  Constant2/1 -> cell_model/1(T)
  Unit Delay/1 -> cell_model/4(zkp)
  cell_model/2(irkc) -> irc1/1, Unit Delay1/1, States/2
  Unit Delay1/1 -> cell_model/5(irkp)
  Constant/1 -> cell_model/3(iR0)

== system sim_battery_pack_simulink_18_11/SCM1/cell7 ==
  ik1 : Inport
  Constant : Constant  Value=R0
  Constant1 : Constant  Value=dt
  Constant2 : Constant  Value=T
  States : Scope  NumInputPorts=2
  Unit Delay : UnitDelay  InitialCondition=Z0(7,1)  SampleTime=-1  HasFrameUpgradeWarning=on
  Unit Delay1 : UnitDelay  SampleTime=-1  HasFrameUpgradeWarning=on
  Voltage : Scope  NumInputPorts=2
  cell_model : MATLAB Function  TreatAsAtomicUnit=on
  V1 : Outport
  Z1 : Outport  Port=2
  irc1 : Outport  Port=3
  wires:
  Constant/1 -> cell_model/3(iR0)
  Unit Delay1/1 -> cell_model/5(irkp)
  cell_model/2(irkc) -> States/2, Unit Delay1/1, irc1/1
  Unit Delay/1 -> cell_model/4(zkp)
  Constant2/1 -> cell_model/1(T)
  Constant1/1 -> cell_model/2(deltaT)
  cell_model/1(vk) -> Voltage/1, V1/1
  cell_model/3(zkc) -> States/1, Unit Delay/1, Z1/1
  ik1/1 -> cell_model/6(ik)
  cell_model/4(OCV) -> Voltage/2

== system sim_battery_pack_simulink_18_11/SCM1/cell8 ==
  ik1 : Inport
  Constant : Constant  Value=R0
  Constant1 : Constant  Value=dt
  Constant2 : Constant  Value=T
  States : Scope  NumInputPorts=2
  Unit Delay : UnitDelay  InitialCondition=Z0(8,1)  SampleTime=-1  HasFrameUpgradeWarning=on
  Unit Delay1 : UnitDelay  SampleTime=-1  HasFrameUpgradeWarning=on
  Voltage : Scope  NumInputPorts=2
  cell_model : MATLAB Function  TreatAsAtomicUnit=on
  V1 : Outport
  Z1 : Outport  Port=2
  irc1 : Outport  Port=3
  wires:
  cell_model/4(OCV) -> Voltage/2
  ik1/1 -> cell_model/6(ik)
  cell_model/3(zkc) -> Z1/1, Unit Delay/1, States/1
  cell_model/1(vk) -> V1/1, Voltage/1
  Constant1/1 -> cell_model/2(deltaT)
  Constant2/1 -> cell_model/1(T)
  Unit Delay/1 -> cell_model/4(zkp)
  cell_model/2(irkc) -> irc1/1, Unit Delay1/1, States/2
  Unit Delay1/1 -> cell_model/5(irkp)
  Constant/1 -> cell_model/3(iR0)

== system sim_battery_pack_simulink_18_11/SCM1/cell9 ==
  ik1 : Inport
  Constant : Constant  Value=R0
  Constant1 : Constant  Value=dt
  Constant2 : Constant  Value=T
  States : Scope  NumInputPorts=2
  Unit Delay : UnitDelay  InitialCondition=Z0(9,1)  SampleTime=-1  HasFrameUpgradeWarning=on
  Unit Delay1 : UnitDelay  SampleTime=-1  HasFrameUpgradeWarning=on
  Voltage : Scope  NumInputPorts=2
  cell_model : MATLAB Function  TreatAsAtomicUnit=on
  V1 : Outport
  Z1 : Outport  Port=2
  irc1 : Outport  Port=3
  wires:
  Constant/1 -> cell_model/3(iR0)
  Unit Delay1/1 -> cell_model/5(irkp)
  cell_model/2(irkc) -> States/2, Unit Delay1/1, irc1/1
  Unit Delay/1 -> cell_model/4(zkp)
  Constant2/1 -> cell_model/1(T)
  Constant1/1 -> cell_model/2(deltaT)
  cell_model/1(vk) -> Voltage/1, V1/1
  cell_model/3(zkc) -> States/1, Unit Delay/1, Z1/1
  ik1/1 -> cell_model/6(ik)
  cell_model/4(OCV) -> Voltage/2

== system sim_battery_pack_simulink_18_11/SCM2/cell1 ==
  ik1 : Inport
  Constant : Constant  Value=R0
  Constant1 : Constant  Value=dt
  Constant2 : Constant  Value=T
  States : Scope  NumInputPorts=2
  Unit Delay : UnitDelay  InitialCondition=Z0(1,2)  SampleTime=-1  HasFrameUpgradeWarning=on
  Unit Delay1 : UnitDelay  SampleTime=-1  HasFrameUpgradeWarning=on
  Voltage : Scope  NumInputPorts=2
  cell_model : MATLAB Function  TreatAsAtomicUnit=on
  V1 : Outport
  Z1 : Outport  Port=2
  irc1 : Outport  Port=3
  wires:
  Constant/1 -> cell_model/3(iR0)
  Unit Delay1/1 -> cell_model/5(irkp)
  cell_model/2(irkc) -> States/2, Unit Delay1/1, irc1/1
  Unit Delay/1 -> cell_model/4(zkp)
  Constant2/1 -> cell_model/1(T)
  Constant1/1 -> cell_model/2(deltaT)
  cell_model/1(vk) -> Voltage/1, V1/1
  cell_model/3(zkc) -> States/1, Unit Delay/1, Z1/1
  ik1/1 -> cell_model/6(ik)
  cell_model/4(OCV) -> Voltage/2

== system sim_battery_pack_simulink_18_11/SCM2/cell10 ==
  ik1 : Inport
  Constant : Constant  Value=R0
  Constant1 : Constant  Value=dt
  Constant2 : Constant  Value=T
  States : Scope  NumInputPorts=2
  Unit Delay : UnitDelay  InitialCondition=Z0(10,2)  SampleTime=-1  HasFrameUpgradeWarning=on
  Unit Delay1 : UnitDelay  SampleTime=-1  HasFrameUpgradeWarning=on
  Voltage : Scope  NumInputPorts=2
  cell_model : MATLAB Function  TreatAsAtomicUnit=on
  V1 : Outport
  Z1 : Outport  Port=2
  irc1 : Outport  Port=3
  wires:
  Constant/1 -> cell_model/3(iR0)
  Unit Delay1/1 -> cell_model/5(irkp)
  cell_model/2(irkc) -> States/2, Unit Delay1/1, irc1/1
  Unit Delay/1 -> cell_model/4(zkp)
  Constant2/1 -> cell_model/1(T)
  Constant1/1 -> cell_model/2(deltaT)
  cell_model/1(vk) -> Voltage/1, V1/1
  cell_model/3(zkc) -> States/1, Unit Delay/1, Z1/1
  ik1/1 -> cell_model/6(ik)
  cell_model/4(OCV) -> Voltage/2

== system sim_battery_pack_simulink_18_11/SCM2/cell11 ==
  ik1 : Inport
  Constant : Constant  Value=R0
  Constant1 : Constant  Value=dt
  Constant2 : Constant  Value=T
  States : Scope  NumInputPorts=2
  Unit Delay : UnitDelay  InitialCondition=Z0(11,2)  SampleTime=-1  HasFrameUpgradeWarning=on
  Unit Delay1 : UnitDelay  SampleTime=-1  HasFrameUpgradeWarning=on
  Voltage : Scope  NumInputPorts=2
  cell_model : MATLAB Function  TreatAsAtomicUnit=on
  V1 : Outport
  Z1 : Outport  Port=2
  irc1 : Outport  Port=3
  wires:
  cell_model/4(OCV) -> Voltage/2
  ik1/1 -> cell_model/6(ik)
  cell_model/3(zkc) -> Z1/1, Unit Delay/1, States/1
  cell_model/1(vk) -> V1/1, Voltage/1
  Constant1/1 -> cell_model/2(deltaT)
  Constant2/1 -> cell_model/1(T)
  Unit Delay/1 -> cell_model/4(zkp)
  cell_model/2(irkc) -> irc1/1, Unit Delay1/1, States/2
  Unit Delay1/1 -> cell_model/5(irkp)
  Constant/1 -> cell_model/3(iR0)

== system sim_battery_pack_simulink_18_11/SCM2/cell12 ==
  ik1 : Inport
  Constant : Constant  Value=R0
  Constant1 : Constant  Value=dt
  Constant2 : Constant  Value=T
  States : Scope  NumInputPorts=2
  Unit Delay : UnitDelay  InitialCondition=Z0(12,2)  SampleTime=-1  HasFrameUpgradeWarning=on
  Unit Delay1 : UnitDelay  SampleTime=-1  HasFrameUpgradeWarning=on
  Voltage : Scope  NumInputPorts=2
  cell_model : MATLAB Function  TreatAsAtomicUnit=on
  V1 : Outport
  Z1 : Outport  Port=2
  irc1 : Outport  Port=3
  wires:
  cell_model/4(OCV) -> Voltage/2
  ik1/1 -> cell_model/6(ik)
  cell_model/3(zkc) -> Z1/1, Unit Delay/1, States/1
  cell_model/1(vk) -> V1/1, Voltage/1
  Constant1/1 -> cell_model/2(deltaT)
  Constant2/1 -> cell_model/1(T)
  Unit Delay/1 -> cell_model/4(zkp)
  cell_model/2(irkc) -> irc1/1, Unit Delay1/1, States/2
  Unit Delay1/1 -> cell_model/5(irkp)
  Constant/1 -> cell_model/3(iR0)

== system sim_battery_pack_simulink_18_11/SCM2/cell2 ==
  ik1 : Inport
  Constant : Constant  Value=R0
  Constant1 : Constant  Value=dt
  Constant2 : Constant  Value=T
  States : Scope  NumInputPorts=2
  Unit Delay : UnitDelay  InitialCondition=Z0(2,2)  SampleTime=-1  HasFrameUpgradeWarning=on
  Unit Delay1 : UnitDelay  SampleTime=-1  HasFrameUpgradeWarning=on
  Voltage : Scope  NumInputPorts=2
  cell_model : MATLAB Function  TreatAsAtomicUnit=on
  V1 : Outport
  Z1 : Outport  Port=2
  irc1 : Outport  Port=3
  wires:
  Constant/1 -> cell_model/3(iR0)
  Unit Delay1/1 -> cell_model/5(irkp)
  cell_model/2(irkc) -> States/2, Unit Delay1/1, irc1/1
  Unit Delay/1 -> cell_model/4(zkp)
  Constant2/1 -> cell_model/1(T)
  Constant1/1 -> cell_model/2(deltaT)
  cell_model/1(vk) -> Voltage/1, V1/1
  cell_model/3(zkc) -> States/1, Unit Delay/1, Z1/1
  ik1/1 -> cell_model/6(ik)
  cell_model/4(OCV) -> Voltage/2

== system sim_battery_pack_simulink_18_11/SCM2/cell3 ==
  ik1 : Inport
  Constant : Constant  Value=R0
  Constant1 : Constant  Value=dt
  Constant2 : Constant  Value=T
  States : Scope  NumInputPorts=2
  Unit Delay : UnitDelay  InitialCondition=Z0(3,2)  SampleTime=-1  HasFrameUpgradeWarning=on
  Unit Delay1 : UnitDelay  SampleTime=-1  HasFrameUpgradeWarning=on
  Voltage : Scope  NumInputPorts=2
  cell_model : MATLAB Function  TreatAsAtomicUnit=on
  V1 : Outport
  Z1 : Outport  Port=2
  irc1 : Outport  Port=3
  wires:
  cell_model/4(OCV) -> Voltage/2
  ik1/1 -> cell_model/6(ik)
  cell_model/3(zkc) -> Z1/1, Unit Delay/1, States/1
  cell_model/1(vk) -> V1/1, Voltage/1
  Constant1/1 -> cell_model/2(deltaT)
  Constant2/1 -> cell_model/1(T)
  Unit Delay/1 -> cell_model/4(zkp)
  cell_model/2(irkc) -> irc1/1, Unit Delay1/1, States/2
  Unit Delay1/1 -> cell_model/5(irkp)
  Constant/1 -> cell_model/3(iR0)

== system sim_battery_pack_simulink_18_11/SCM2/cell4 ==
  ik1 : Inport
  Constant : Constant  Value=R0
  Constant1 : Constant  Value=dt
  Constant2 : Constant  Value=T
  States : Scope  NumInputPorts=2
  Unit Delay : UnitDelay  InitialCondition=Z0(4,2)  SampleTime=-1  HasFrameUpgradeWarning=on
  Unit Delay1 : UnitDelay  SampleTime=-1  HasFrameUpgradeWarning=on
  Voltage : Scope  NumInputPorts=2
  cell_model : MATLAB Function  TreatAsAtomicUnit=on
  V1 : Outport
  Z1 : Outport  Port=2
  irc1 : Outport  Port=3
  wires:
  cell_model/4(OCV) -> Voltage/2
  ik1/1 -> cell_model/6(ik)
  cell_model/3(zkc) -> Z1/1, Unit Delay/1, States/1
  cell_model/1(vk) -> V1/1, Voltage/1
  Constant1/1 -> cell_model/2(deltaT)
  Constant2/1 -> cell_model/1(T)
  Unit Delay/1 -> cell_model/4(zkp)
  cell_model/2(irkc) -> irc1/1, Unit Delay1/1, States/2
  Unit Delay1/1 -> cell_model/5(irkp)
  Constant/1 -> cell_model/3(iR0)

== system sim_battery_pack_simulink_18_11/SCM2/cell5 ==
  ik1 : Inport
  Constant : Constant  Value=R0
  Constant1 : Constant  Value=dt
  Constant2 : Constant  Value=T
  States : Scope  NumInputPorts=2
  Unit Delay : UnitDelay  InitialCondition=Z0(5,2)  SampleTime=-1  HasFrameUpgradeWarning=on
  Unit Delay1 : UnitDelay  SampleTime=-1  HasFrameUpgradeWarning=on
  Voltage : Scope  NumInputPorts=2
  cell_model : MATLAB Function  TreatAsAtomicUnit=on
  V1 : Outport
  Z1 : Outport  Port=2
  irc1 : Outport  Port=3
  wires:
  Constant/1 -> cell_model/3(iR0)
  Unit Delay1/1 -> cell_model/5(irkp)
  cell_model/2(irkc) -> States/2, Unit Delay1/1, irc1/1
  Unit Delay/1 -> cell_model/4(zkp)
  Constant2/1 -> cell_model/1(T)
  Constant1/1 -> cell_model/2(deltaT)
  cell_model/1(vk) -> Voltage/1, V1/1
  cell_model/3(zkc) -> States/1, Unit Delay/1, Z1/1
  ik1/1 -> cell_model/6(ik)
  cell_model/4(OCV) -> Voltage/2

== system sim_battery_pack_simulink_18_11/SCM2/cell6 ==
  ik1 : Inport
  Constant : Constant  Value=R0
  Constant1 : Constant  Value=dt
  Constant2 : Constant  Value=T
  States : Scope  NumInputPorts=2
  Unit Delay : UnitDelay  InitialCondition=Z0(6,2)  SampleTime=-1  HasFrameUpgradeWarning=on
  Unit Delay1 : UnitDelay  SampleTime=-1  HasFrameUpgradeWarning=on
  Voltage : Scope  NumInputPorts=2
  cell_model : MATLAB Function  TreatAsAtomicUnit=on
  V1 : Outport
  Z1 : Outport  Port=2
  irc1 : Outport  Port=3
  wires:
  Constant/1 -> cell_model/3(iR0)
  Unit Delay1/1 -> cell_model/5(irkp)
  cell_model/2(irkc) -> States/2, Unit Delay1/1, irc1/1
  Unit Delay/1 -> cell_model/4(zkp)
  Constant2/1 -> cell_model/1(T)
  Constant1/1 -> cell_model/2(deltaT)
  cell_model/1(vk) -> Voltage/1, V1/1
  cell_model/3(zkc) -> States/1, Unit Delay/1, Z1/1
  ik1/1 -> cell_model/6(ik)
  cell_model/4(OCV) -> Voltage/2

== system sim_battery_pack_simulink_18_11/SCM2/cell7 ==
  ik1 : Inport
  Constant : Constant  Value=R0
  Constant1 : Constant  Value=dt
  Constant2 : Constant  Value=T
  States : Scope  NumInputPorts=2
  Unit Delay : UnitDelay  InitialCondition=Z0(7,2)  SampleTime=-1  HasFrameUpgradeWarning=on
  Unit Delay1 : UnitDelay  SampleTime=-1  HasFrameUpgradeWarning=on
  Voltage : Scope  NumInputPorts=2
  cell_model : MATLAB Function  TreatAsAtomicUnit=on
  V1 : Outport
  Z1 : Outport  Port=2
  irc1 : Outport  Port=3
  wires:
  cell_model/4(OCV) -> Voltage/2
  ik1/1 -> cell_model/6(ik)
  cell_model/3(zkc) -> Z1/1, Unit Delay/1, States/1
  cell_model/1(vk) -> V1/1, Voltage/1
  Constant1/1 -> cell_model/2(deltaT)
  Constant2/1 -> cell_model/1(T)
  Unit Delay/1 -> cell_model/4(zkp)
  cell_model/2(irkc) -> irc1/1, Unit Delay1/1, States/2
  Unit Delay1/1 -> cell_model/5(irkp)
  Constant/1 -> cell_model/3(iR0)

== system sim_battery_pack_simulink_18_11/SCM2/cell8 ==
  ik1 : Inport
  Constant : Constant  Value=R0
  Constant1 : Constant  Value=dt
  Constant2 : Constant  Value=T
  States : Scope  NumInputPorts=2
  Unit Delay : UnitDelay  InitialCondition=Z0(8,2)  SampleTime=-1  HasFrameUpgradeWarning=on
  Unit Delay1 : UnitDelay  SampleTime=-1  HasFrameUpgradeWarning=on
  Voltage : Scope  NumInputPorts=2
  cell_model : MATLAB Function  TreatAsAtomicUnit=on
  V1 : Outport
  Z1 : Outport  Port=2
  irc1 : Outport  Port=3
  wires:
  Constant/1 -> cell_model/3(iR0)
  Unit Delay1/1 -> cell_model/5(irkp)
  cell_model/2(irkc) -> States/2, Unit Delay1/1, irc1/1
  Unit Delay/1 -> cell_model/4(zkp)
  Constant2/1 -> cell_model/1(T)
  Constant1/1 -> cell_model/2(deltaT)
  cell_model/1(vk) -> Voltage/1, V1/1
  cell_model/3(zkc) -> States/1, Unit Delay/1, Z1/1
  ik1/1 -> cell_model/6(ik)
  cell_model/4(OCV) -> Voltage/2

== system sim_battery_pack_simulink_18_11/SCM2/cell9 ==
  ik1 : Inport
  Constant : Constant  Value=R0
  Constant1 : Constant  Value=dt
  Constant2 : Constant  Value=T
  States : Scope  NumInputPorts=2
  Unit Delay : UnitDelay  InitialCondition=Z0(9,2)  SampleTime=-1  HasFrameUpgradeWarning=on
  Unit Delay1 : UnitDelay  SampleTime=-1  HasFrameUpgradeWarning=on
  Voltage : Scope  NumInputPorts=2
  cell_model : MATLAB Function  TreatAsAtomicUnit=on
  V1 : Outport
  Z1 : Outport  Port=2
  irc1 : Outport  Port=3
  wires:
  cell_model/4(OCV) -> Voltage/2
  ik1/1 -> cell_model/6(ik)
  cell_model/3(zkc) -> Z1/1, Unit Delay/1, States/1
  cell_model/1(vk) -> V1/1, Voltage/1
  Constant1/1 -> cell_model/2(deltaT)
  Constant2/1 -> cell_model/1(T)
  Unit Delay/1 -> cell_model/4(zkp)
  cell_model/2(irkc) -> irc1/1, Unit Delay1/1, States/2
  Unit Delay1/1 -> cell_model/5(irkp)
  Constant/1 -> cell_model/3(iR0)

== system sim_battery_pack_simulink_18_11/SCM3/cell1 ==
  ik1 : Inport
  Constant : Constant  Value=R0
  Constant1 : Constant  Value=dt
  Constant2 : Constant  Value=T
  States : Scope  NumInputPorts=2
  Unit Delay : UnitDelay  InitialCondition=Z0(1,3)  SampleTime=-1  HasFrameUpgradeWarning=on
  Unit Delay1 : UnitDelay  SampleTime=-1  HasFrameUpgradeWarning=on
  Voltage : Scope  NumInputPorts=2
  cell_model : MATLAB Function  TreatAsAtomicUnit=on
  V1 : Outport
  Z1 : Outport  Port=2
  irc1 : Outport  Port=3
  wires:
  cell_model/4(OCV) -> Voltage/2
  ik1/1 -> cell_model/6(ik)
  cell_model/3(zkc) -> Z1/1, Unit Delay/1, States/1
  cell_model/1(vk) -> V1/1, Voltage/1
  Constant1/1 -> cell_model/2(deltaT)
  Constant2/1 -> cell_model/1(T)
  Unit Delay/1 -> cell_model/4(zkp)
  cell_model/2(irkc) -> irc1/1, Unit Delay1/1, States/2
  Unit Delay1/1 -> cell_model/5(irkp)
  Constant/1 -> cell_model/3(iR0)

== system sim_battery_pack_simulink_18_11/SCM3/cell10 ==
  ik1 : Inport
  Constant : Constant  Value=R0
  Constant1 : Constant  Value=dt
  Constant2 : Constant  Value=T
  States : Scope  NumInputPorts=2
  Unit Delay : UnitDelay  InitialCondition=Z0(10,3)  SampleTime=-1  HasFrameUpgradeWarning=on
  Unit Delay1 : UnitDelay  SampleTime=-1  HasFrameUpgradeWarning=on
  Voltage : Scope  NumInputPorts=2
  cell_model : MATLAB Function  TreatAsAtomicUnit=on
  V1 : Outport
  Z1 : Outport  Port=2
  irc1 : Outport  Port=3
  wires:
  cell_model/4(OCV) -> Voltage/2
  ik1/1 -> cell_model/6(ik)
  cell_model/3(zkc) -> Z1/1, Unit Delay/1, States/1
  cell_model/1(vk) -> V1/1, Voltage/1
  Constant1/1 -> cell_model/2(deltaT)
  Constant2/1 -> cell_model/1(T)
  Unit Delay/1 -> cell_model/4(zkp)
  cell_model/2(irkc) -> irc1/1, Unit Delay1/1, States/2
  Unit Delay1/1 -> cell_model/5(irkp)
  Constant/1 -> cell_model/3(iR0)

== system sim_battery_pack_simulink_18_11/SCM3/cell11 ==
  ik1 : Inport
  Constant : Constant  Value=R0
  Constant1 : Constant  Value=dt
  Constant2 : Constant  Value=T
  States : Scope  NumInputPorts=2
  Unit Delay : UnitDelay  InitialCondition=Z0(11,3)  SampleTime=-1  HasFrameUpgradeWarning=on
  Unit Delay1 : UnitDelay  SampleTime=-1  HasFrameUpgradeWarning=on
  Voltage : Scope  NumInputPorts=2
  cell_model : MATLAB Function  TreatAsAtomicUnit=on
  V1 : Outport
  Z1 : Outport  Port=2
  irc1 : Outport  Port=3
  wires:
  Constant/1 -> cell_model/3(iR0)
  Unit Delay1/1 -> cell_model/5(irkp)
  cell_model/2(irkc) -> States/2, Unit Delay1/1, irc1/1
  Unit Delay/1 -> cell_model/4(zkp)
  Constant2/1 -> cell_model/1(T)
  Constant1/1 -> cell_model/2(deltaT)
  cell_model/1(vk) -> Voltage/1, V1/1
  cell_model/3(zkc) -> States/1, Unit Delay/1, Z1/1
  ik1/1 -> cell_model/6(ik)
  cell_model/4(OCV) -> Voltage/2

== system sim_battery_pack_simulink_18_11/SCM3/cell12 ==
  ik1 : Inport
  Constant : Constant  Value=R0
  Constant1 : Constant  Value=dt
  Constant2 : Constant  Value=T
  States : Scope  NumInputPorts=2
  Unit Delay : UnitDelay  InitialCondition=Z0(12,3)  SampleTime=-1  HasFrameUpgradeWarning=on
  Unit Delay1 : UnitDelay  SampleTime=-1  HasFrameUpgradeWarning=on
  Voltage : Scope  NumInputPorts=2
  cell_model : MATLAB Function  TreatAsAtomicUnit=on
  V1 : Outport
  Z1 : Outport  Port=2
  irc1 : Outport  Port=3
  wires:
  Constant/1 -> cell_model/3(iR0)
  Unit Delay1/1 -> cell_model/5(irkp)
  cell_model/2(irkc) -> States/2, Unit Delay1/1, irc1/1
  Unit Delay/1 -> cell_model/4(zkp)
  Constant2/1 -> cell_model/1(T)
  Constant1/1 -> cell_model/2(deltaT)
  cell_model/1(vk) -> Voltage/1, V1/1
  cell_model/3(zkc) -> States/1, Unit Delay/1, Z1/1
  ik1/1 -> cell_model/6(ik)
  cell_model/4(OCV) -> Voltage/2
